simulink model "MotorCtrl_FOC_Math"  (R2025b)
settings: Solver=FixedStepDiscrete  StartTime=0.0  StopTime=5  FixedStep=MC_Sim_BaseStep  RelTol=1e-3  EnableMultiTasking=on
values from neighbouring files (symbols this model uses):
  MC_ADC_BitNum = 0.0    [MotorControlDataDictionary_Math.sldd]
  MC_ADC_Offset = 0.0    [MotorControlDataDictionary_Math.sldd]
  MC_ADC_VRef = 1.0    [MotorControlDataDictionary_Math.sldd]
  MC_CSA_Gain = 1.0    [MotorControlDataDictionary_Math.sldd]
  MC_MOS_DeadTime = 1.3E-6    [MotorControlDataDictionary_Math.sldd]
  MC_Motor_Mechinal_Damp = 1.0E-5    [MotorControlDataDictionary_Math.sldd]
  MC_Motor_Mechinal_Fric = 0.0    [MotorControlDataDictionary_Math.sldd]
  MC_Motor_Mechinal_Inertia = 0.0103    [MotorControlDataDictionary_Math.sldd]
  MC_Motor_Phi = 0.0059190254913385806    [MotorControlDataDictionary_Math.sldd]
  MC_Motor_Rotor_Pn = 4.0    [MotorControlDataDictionary_Math.sldd]
  MC_Motor_Stator_Ld = 5.6345E-5    [MotorControlDataDictionary_Math.sldd]
  MC_Motor_Stator_Lq = 5.6345E-5    [MotorControlDataDictionary_Math.sldd]
  MC_Motor_Stator_Rs = 0.0286    [MotorControlDataDictionary_Math.sldd]
  MC_Param_CurrentPI_Ki = 0.0089705790612839825    [MotorControlDataDictionary_Math.sldd]
  MC_Param_CurrentPI_Kp = 0.283220860906427    [MotorControlDataDictionary_Math.sldd]
  MC_Param_CurrentPI_UdInteMax = 7.794228634059948    [MotorControlDataDictionary_Math.sldd]
  MC_Param_CurrentPI_UdInteMin = -7.794228634059948    [MotorControlDataDictionary_Math.sldd]
  MC_Param_CurrentPI_UdMax = 7.794228634059948    [MotorControlDataDictionary_Math.sldd]
  MC_Param_CurrentPI_UdMin = -7.794228634059948    [MotorControlDataDictionary_Math.sldd]
  MC_Param_CurrentPI_UqInteMax = 7.794228634059948    [MotorControlDataDictionary_Math.sldd]
  MC_Param_CurrentPI_UqInteMin = -7.794228634059948    [MotorControlDataDictionary_Math.sldd]
  MC_Param_CurrentPI_UqMax = 7.794228634059948    [MotorControlDataDictionary_Math.sldd]
  MC_Param_CurrentPI_UqMin = -7.794228634059948    [MotorControlDataDictionary_Math.sldd]
  MC_Param_Flux_Gamma = 750000.0    [MotorControlDataDictionary_Math.sldd]
  MC_Param_Flux_Lalpha = 5.6345E-5    [MotorControlDataDictionary_Math.sldd]
  MC_Param_Flux_Lbeta = 5.6345E-5    [MotorControlDataDictionary_Math.sldd]
  MC_Param_Flux_Ralpha = 0.0286    [MotorControlDataDictionary_Math.sldd]
  MC_Param_Flux_Rbeta = 0.0286    [MotorControlDataDictionary_Math.sldd]
  MC_Param_Luen_BEMFalpha = -17747.803709290976    [MotorControlDataDictionary_Math.sldd]
  MC_Param_Luen_BEMFbeta = -17747.803709290976    [MotorControlDataDictionary_Math.sldd]
  MC_Param_Luen_BEMFErr = 10.0    [MotorControlDataDictionary_Math.sldd]
  MC_Param_Luen_Currentalpha = -507.58718608572195    [MotorControlDataDictionary_Math.sldd]
  MC_Param_Luen_Currentbeta = -507.58718608572195    [MotorControlDataDictionary_Math.sldd]
  MC_Param_Luen_CurrentErr = 400.0    [MotorControlDataDictionary_Math.sldd]
  MC_Param_Luen_PLL_Ki = 0.24634532585119037    [MotorControlDataDictionary_Math.sldd]
  MC_Param_Luen_PLL_Kp = 125.66370614359172    [MotorControlDataDictionary_Math.sldd]
  MC_Param_Luen_Voltagealpha = 17747.803709290976    [MotorControlDataDictionary_Math.sldd]
  MC_Param_Luen_Voltagebeta = 17747.803709290976    [MotorControlDataDictionary_Math.sldd]
  MC_Param_PhasetoReal = 500.0    [MotorControlDataDictionary_Math.sldd]
  MC_Param_SMO_CoffA = 0.968326559588251    [MotorControlDataDictionary_Math.sldd]
  MC_Param_SMO_CoffB = 1.1074629514597569    [MotorControlDataDictionary_Math.sldd]
  MC_Param_SpeedCtrl_IdMax = 60.0    [MotorControlDataDictionary_Math.sldd]
  MC_Param_SpeedCtrl_IdMin = -60.0    [MotorControlDataDictionary_Math.sldd]
  MC_Param_SpeedCtrl_IqMax = 60.0    [MotorControlDataDictionary_Math.sldd]
  MC_Param_SpeedCtrl_IqMin = -60.0    [MotorControlDataDictionary_Math.sldd]
  MC_Param_SpeedPI_Ki = 0.57157085739428382    [MotorControlDataDictionary_Math.sldd]
  MC_Param_SpeedPI_Kp = 9.1114109857344836    [MotorControlDataDictionary_Math.sldd]
  MC_Param_SpeedtoTheta = 6.24E-5    [MotorControlDataDictionary_Math.sldd]
  MC_Param_SVPWM_DutyMax = 0.98    [MotorControlDataDictionary_Math.sldd]
  MC_Param_SVPWM_DutyMin = 0.02    [MotorControlDataDictionary_Math.sldd]
  MC_Param_SVPWM_SampleOffset1 = 0.02    [MotorControlDataDictionary_Math.sldd]
  MC_Param_SVPWM_SampleOffset2 = 0.015    [MotorControlDataDictionary_Math.sldd]
  MC_Param_SVPWM_SampleValid = 0.0096153846153846159    [MotorControlDataDictionary_Math.sldd]
  MC_Param_Zero = 0.0    [MotorControlDataDictionary_Math.sldd]
  MC_Sample_CurrentNoise = 1.0E-15    [MotorControlDataDictionary_Math.sldd]
  MC_Sample_Rs = 0.002    [MotorControlDataDictionary_Math.sldd]
  MC_Sample_VbusNoise = 1.0E-15    [MotorControlDataDictionary_Math.sldd]
  MC_Sim_BaseStep = 2.08E-8    [MotorControlDataDictionary_Math.sldd]
  MC_Sim_HFTStep = 6.24E-5    [MotorControlDataDictionary_Math.sldd]
  MC_Sim_MFTStep = 0.0019968    [MotorControlDataDictionary_Math.sldd]
libraries: simulink x28, nesl_utility x19, fl_lib x14, ee_lib x13, autolibpmsminterior x2, autolibinverter x1
(part 8 of 8)

== system MotorCtrl_FOC_Math/MFTask/adrcofSpeed/LESO/falFunc1 ==
  Err : Inport
  Alpha : Inport  Port=2
  Delta : Inport  Port=3
  Abs : Abs  SaturateOnIntegerOverflow=off
  Constant : Constant  OutDataTypeStr=single
  Divide : Product  Inputs=*/  OutDataTypeStr=single  RndMeth=Simplest
  Math Function : Math  Operator=pow  OutputSignalType=real
  Math Function1 : Math  Operator=pow  OutputSignalType=real
  Product : Product  OutDataTypeStr=single  RndMeth=Simplest
  Relational Operator : RelationalOperator  Operator=<=  OutDataTypeStr=boolean  RndMeth=Simplest  InputSameDT=off
  Sign : Signum
  Subtract : Sum  Inputs=+-
  Switch : Switch  Criteria=u2 > Threshold  SaturateOnIntegerOverflow=off  InputSameDT=off
  FalOutput : Outport
  wires:
  Switch/1 -> FalOutput/1
  Product/1 -> Switch/3
  Sign/1 -> Product/2
  Math Function1/1 -> Product/1
  Alpha/1 -> Subtract/2, Math Function1/2
  Divide/1 -> Switch/1
  Constant/1 -> Subtract/1
  Subtract/1 -> Math Function/2
  Math Function/1 -> Divide/2
  Relational Operator/1 -> Switch/2
  Delta/1 -> Relational Operator/2, Math Function/1
  Abs/1 -> Relational Operator/1, Math Function1/1
  Err/1 -> Abs/1, Sign/1, Divide/1

== system MotorCtrl_FOC_Math/MFTask/adrcofSpeed/LESO/falFunc2 ==
  Err : Inport
  Alpha : Inport  Port=2
  Delta : Inport  Port=3
  Abs : Abs  SaturateOnIntegerOverflow=off
  Constant : Constant  OutDataTypeStr=single
  Divide : Product  Inputs=*/  OutDataTypeStr=single  RndMeth=Simplest
  Math Function : Math  Operator=pow  OutputSignalType=real
  Math Function1 : Math  Operator=pow  OutputSignalType=real
  Product : Product  OutDataTypeStr=single  RndMeth=Simplest
  Relational Operator : RelationalOperator  Operator=<=  OutDataTypeStr=boolean  RndMeth=Simplest  InputSameDT=off
  Sign : Signum
  Subtract : Sum  Inputs=+-
  Switch : Switch  Criteria=u2 > Threshold  SaturateOnIntegerOverflow=off  InputSameDT=off
  FalOutput : Outport
  wires:
  Switch/1 -> FalOutput/1
  Product/1 -> Switch/3
  Sign/1 -> Product/2
  Math Function1/1 -> Product/1
  Alpha/1 -> Subtract/2, Math Function1/2
  Divide/1 -> Switch/1
  Constant/1 -> Subtract/1
  Subtract/1 -> Math Function/2
  Math Function/1 -> Divide/2
  Relational Operator/1 -> Switch/2
  Delta/1 -> Relational Operator/2, Math Function/1
  Abs/1 -> Relational Operator/1, Math Function1/1
  Err/1 -> Abs/1, Sign/1, Divide/1

== system MotorCtrl_FOC_Math/MFTask/adrcofSpeed/LESO/falFunc3 ==
  Err : Inport
  Alpha : Inport  Port=2
  Delta : Inport  Port=3
  Abs : Abs  SaturateOnIntegerOverflow=off
  Constant : Constant  OutDataTypeStr=single
  Divide : Product  Inputs=*/  OutDataTypeStr=single  RndMeth=Simplest
  Math Function : Math  Operator=pow  OutputSignalType=real
  Math Function1 : Math  Operator=pow  OutputSignalType=real
  Product : Product  OutDataTypeStr=single  RndMeth=Simplest
  Relational Operator : RelationalOperator  Operator=<=  OutDataTypeStr=boolean  RndMeth=Simplest  InputSameDT=off
  Sign : Signum
  Subtract : Sum  Inputs=+-
  Switch : Switch  Criteria=u2 > Threshold  SaturateOnIntegerOverflow=off  InputSameDT=off
  FalOutput : Outport
  wires:
  Err/1 -> Divide/1, Sign/1, Abs/1
  Abs/1 -> Math Function1/1, Relational Operator/1
  Delta/1 -> Math Function/1, Relational Operator/2
  Relational Operator/1 -> Switch/2
  Math Function/1 -> Divide/2
  Subtract/1 -> Math Function/2
  Constant/1 -> Subtract/1
  Divide/1 -> Switch/1
  Alpha/1 -> Math Function1/2, Subtract/2
  Math Function1/1 -> Product/1
  Sign/1 -> Product/2
  Product/1 -> Switch/3
  Switch/1 -> FalOutput/1

== system MotorCtrl_FOC_Math/MFTask/adrcofSpeed/NLSEF/Subsystem ==
  In1 : Inport
  Gain : Gain  Gain=0.05
  IqRef : Outport
  wires:
  In1/1 -> Gain/1
  Gain/1 -> IqRef/1

== system MotorCtrl_FOC_Math/MFTask/adrcofSpeed/Tracking-Differentiator/Subsystem ==
  Ref_In : Inport
  X1 : Inport  Port=2
  X2 : Inport  Port=3
  Abs : Abs  SaturateOnIntegerOverflow=off
  Abs1 : Abs  SaturateOnIntegerOverflow=off
  Add : Sum
  Add1 : Sum
  Add2 : Sum  Inputs=-+
  Constant : Constant  Value=100  OutDataTypeStr=single
  Gain : Gain  Gain=MC_Sim_MFTStep  ParamDataTypeStr=single  OutDataTypeStr=single  RndMeth=Simplest
  Gain1 : Gain  Gain=MC_Sim_MFTStep  ParamDataTypeStr=single  OutDataTypeStr=single  RndMeth=Simplest
  Gain2 : Gain  Gain=MC_Sim_MFTStep  ParamDataTypeStr=single  OutDataTypeStr=single  RndMeth=Simplest
  Gain3 : Gain  Gain=8  ParamDataTypeStr=single  OutDataTypeStr=single  RndMeth=Simplest
  Gain4 : Gain  Gain=1/2  ParamDataTypeStr=single  OutDataTypeStr=single  RndMeth=Simplest
  Gain5 : Gain  Gain=1/MC_Sim_MFTStep  ParamDataTypeStr=single  OutDataTypeStr=single  RndMeth=Simplest
  Gain6 : Gain
  Gain7 : Gain  Gain=1/MC_Sim_MFTStep  ParamDataTypeStr=single  OutDataTypeStr=single  RndMeth=Simplest
  Gain8 : Gain  Gain=-1  ParamDataTypeStr=single  OutDataTypeStr=single  RndMeth=Simplest
  Product : Product  OutDataTypeStr=single  RndMeth=Simplest
  Product1 : Product
  Product2 : Product
  Relational Operator : RelationalOperator  Operator=>  OutDataTypeStr=boolean  RndMeth=Simplest  InputSameDT=off
  Relational Operator1 : RelationalOperator  OutDataTypeStr=boolean  RndMeth=Simplest  InputSameDT=off
  Sign : Signum
  Sign1 : Signum
  Sqrt : Sqrt
  Square : Math  Operator=square
  Subtract : Sum  Inputs=+-
  Subtract1 : Sum  Inputs=+-
  Switch : Switch  Criteria=u2 > Threshold  OutDataTypeStr=single  RndMeth=Simplest  SaturateOnIntegerOverflow=off  InputSameDT=off
  Switch1 : Switch  Criteria=u2 > Threshold  OutDataTypeStr=single  RndMeth=Simplest  SaturateOnIntegerOverflow=off  InputSameDT=off
  Ref_TD : Outport
  wires:
  X2/1 -> [x2]
  Ref_In/1 -> [Ref_In]
  X1/1 -> [x1]
  [x2] -> Gain/1
  Gain/1 -> Add/2
  [e] -> Add/1
  Add/1 -> [y]  "y"
  Subtract/1 -> [e]  "e"
  Constant/1 -> Gain3/1, Product1/2, Gain1/1  "r"
  Gain1/1 -> Gain2/1, [d]  "d"
  Gain2/1 -> [d0]  "d0"
  [y] -> Abs/1
  Abs/1 -> Relational Operator/1, Sign1/1, Product/2
  Gain3/1 -> Product/1
  [d] -> Subtract1/2, Square/1
  Product/1 -> Add1/1
  Square/1 -> Add1/2
  Add1/1 -> Sqrt/1
  [d0] -> Relational Operator/2
  Relational Operator/1 -> Switch/2
  Switch/1 -> Add2/1
  [x2] -> Add2/2
  [a0] -> Subtract1/1
  Subtract1/1 -> Gain4/1
  Gain4/1 -> Switch/1
  [y] -> Gain5/1
  Gain5/1 -> Switch/3
  Add2/1 -> [a]  "a"
  Abs1/1 -> Relational Operator1/1
  [d] -> Relational Operator1/2
  Relational Operator1/1 -> Switch1/2
  Switch1/1 -> Gain8/1  "Ref_TD"
  [a] -> Gain7/1, Sign/1, Abs1/1
  Gain7/1 -> Switch1/1
  Sign/1 -> Product1/1
  Product1/1 -> Switch1/3
  Gain8/1 -> Ref_TD/1  "N_Ref_TD"
  [x1] -> Subtract/1
  [Ref_In] -> Subtract/2
  Sign1/1 -> Gain6/1
  Sqrt/1 -> Product2/1  "a0"
  Product2/1 -> [a0]
  Gain6/1 -> Product2/2
